simulink model "test"  (R2022b)
settings: Solver=ode8  StartTime=0.0  StopTime=0.01  FixedStep=1e-5  RelTol=1e-3
settings Model: Creator=isaac  LastModifiedBy=isaac

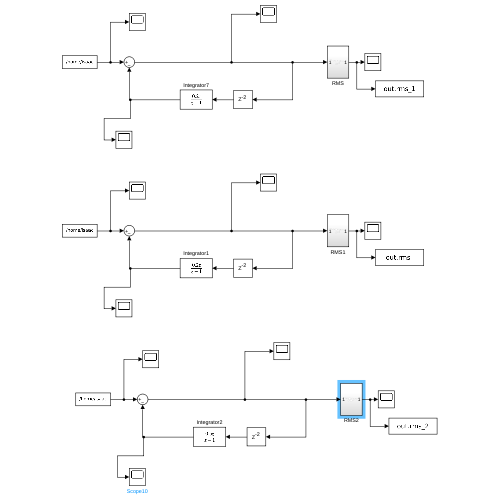
[thumbnail: Simulink's stored preview of the top-level diagram]
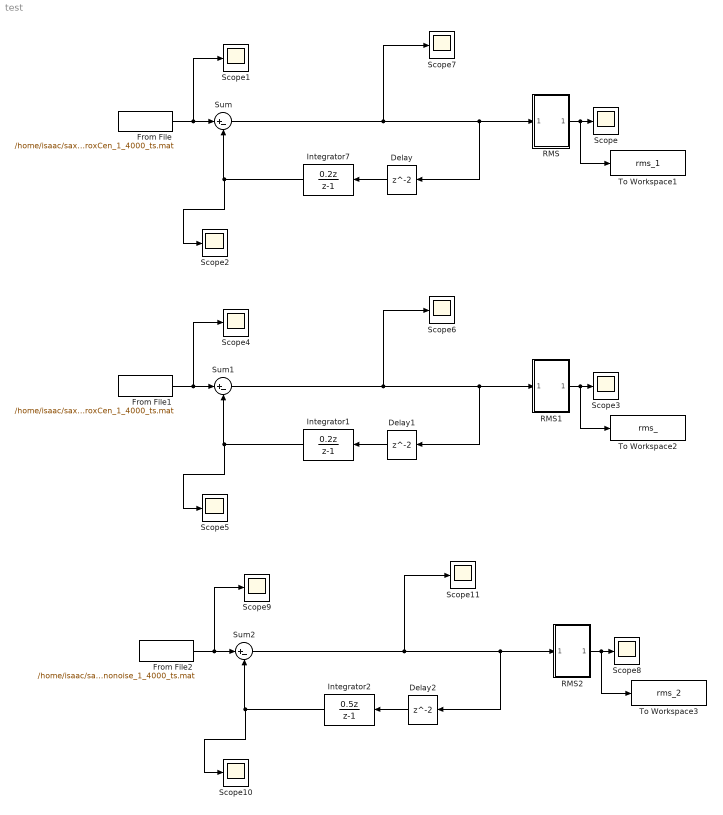
== system test ==
  Delay : Delay  SampleTime=0.001
  Delay1 : Delay  SampleTime=0.001
  Delay2 : Delay  SampleTime=0.001
  From File : FromFile  FileName=/home/isaac/saxo-plus/Data-Driven-Control-for-AO/DM_dyn/simulink/single_mode_dist_ProxCen_1_4000_ts.mat  SampleTime=0.00025
  From File1 : FromFile  FileName=/home/isaac/saxo-plus/Data-Driven-Control-for-AO/DM_dyn/simulink/single_mode_dist_ProxCen_1_4000_ts.mat  SampleTime=0.001
  From File2 : FromFile  FileName=/home/isaac/saxo-plus/Data-Driven-Control-for-AO/DM_dyn/simulink/single_mode_dist_nonoise_1_4000_ts.mat  SampleTime=0.00025
  Integrator1 : DiscreteTransferFcn  Numerator=[0.2 0]  Denominator=[1 -1]  SampleTime=0.001
  Integrator2 : DiscreteTransferFcn  Numerator=[0.5 0]  Denominator=[1 -1]  SampleTime=0.001
  Integrator7 : DiscreteTransferFcn  Numerator=[0.2 0]  Denominator=[1 -1]  SampleTime=0.001
  RMS : Subsystem
  RMS1 : Subsystem
  RMS2 : Subsystem
  Scope{,1..11} (12 alike) : Scope
  Sum : Sum  Inputs=|+-
  Sum1 : Sum  Inputs=|+-
  Sum2 : Sum  Inputs=|+-
  To Workspace1 : ToWorkspace  VariableName=rms_1  SampleTime=-1
      settings: MaxDataPoints=1
  To Workspace2 : ToWorkspace  VariableName=rms_  SampleTime=-1
      settings: MaxDataPoints=1
  To Workspace3 : ToWorkspace  VariableName=rms_2  SampleTime=-1
      settings: MaxDataPoints=1
  wires:
  Delay/1 -> Integrator7/1
  RMS/1(Out1) -> To Workspace1/1, Scope/1
  Sum/1 -> Scope7/1, Delay/1, RMS/1(In1)
  Integrator7/1 -> Scope2/1, Sum/2
  From File/1 -> Scope1/1, Sum/1
  Sum1/1 -> Scope6/1, Delay1/1, RMS1/1(In1)
  Integrator1/1 -> Scope5/1, Sum1/2
  RMS1/1(Out1) -> To Workspace2/1, Scope3/1
  Delay1/1 -> Integrator1/1
  From File1/1 -> Scope4/1, Sum1/1
  Integrator2/1 -> Scope10/1, Sum2/2
  Sum2/1 -> Scope11/1, Delay2/1, RMS2/1(In1)
  Delay2/1 -> Integrator2/1
  RMS2/1(Out1) -> To Workspace3/1, Scope8/1
  From File2/1 -> Scope9/1, Sum2/1

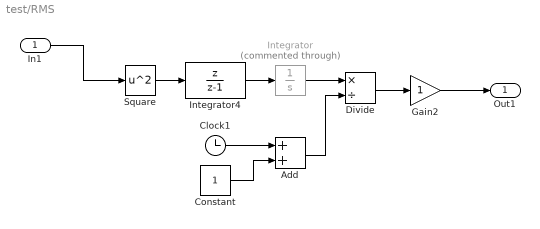
== system test/RMS ==
  In1 : Inport
  Add : Sum
  Clock1 : Clock
  Constant : Constant
  Divide : Product  Inputs=*/
  Gain2 : Gain
  Integrator : Integrator  Commented=through
  Integrator4 : DiscreteTransferFcn  Numerator=[1 0]  Denominator=[1 -1]  SampleTime=0.00025
  Square : Math  Operator=square
  Out1 : Outport
  wires:
  Divide/1 -> Gain2/1
  Integrator4/1 -> Integrator/1
  Square/1 -> Integrator4/1
  In1/1 -> Square/1
  Gain2/1 -> Out1/1
  Add/1 -> Divide/2
  Clock1/1 -> Add/1
  Constant/1 -> Add/2
  Integrator/1 -> Divide/1

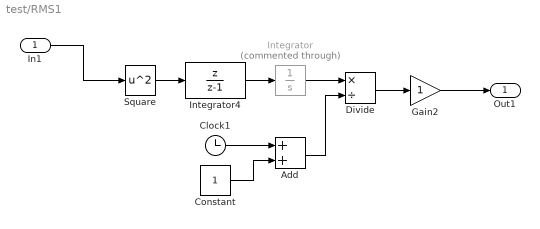
== system test/RMS1 ==
  In1 : Inport
  Add : Sum
  Clock1 : Clock
  Constant : Constant
  Divide : Product  Inputs=*/
  Gain2 : Gain
  Integrator : Integrator  Commented=through
  Integrator4 : DiscreteTransferFcn  Numerator=[1 0]  Denominator=[1 -1]  SampleTime=0.001
  Square : Math  Operator=square
  Out1 : Outport
  wires:
  Divide/1 -> Gain2/1
  Integrator4/1 -> Integrator/1
  Square/1 -> Integrator4/1
  In1/1 -> Square/1
  Gain2/1 -> Out1/1
  Add/1 -> Divide/2
  Clock1/1 -> Add/1
  Constant/1 -> Add/2
  Integrator/1 -> Divide/1

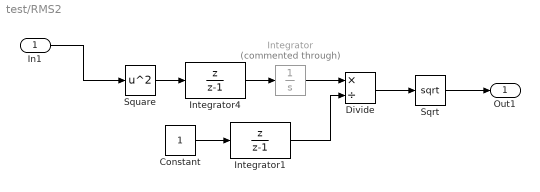
== system test/RMS2 ==
  In1 : Inport
  Constant : Constant
  Divide : Product  Inputs=*/
  Integrator : Integrator  Commented=through
  Integrator1 : DiscreteTransferFcn  Numerator=[1 0]  Denominator=[1 -1]  SampleTime=0.001
  Integrator4 : DiscreteTransferFcn  Numerator=[1 0]  Denominator=[1 -1]  SampleTime=0.001
  Sqrt : Sqrt
  Square : Math  Operator=square
  Out1 : Outport
  wires:
  Integrator4/1 -> Integrator/1
  Square/1 -> Integrator4/1
  In1/1 -> Square/1
  Sqrt/1 -> Out1/1
  Constant/1 -> Integrator1/1
  Integrator/1 -> Divide/1
  Integrator1/1 -> Divide/2
  Divide/1 -> Sqrt/1
